simulink model "CHB1"  (R2014b)
settings: Solver=ode23tb  StartTime=0.0  StopTime=0.57  MaxStep=0.0001  RelTol=1e-3
libraries: powerlib x33, RCTblocks x1
settings Model: Creator=selva  LastModifiedBy=SELVA
settings DataIOCC: SignalLoggingSaveFormat=ModelDataLogs
settings OptimizationCC: ExpressionDepthLimit=2147483647
settings DebuggingCC: UnderspecifiedInitializationDetection=Classic  MergeDetectMultiDrivingBlocksExec=none  FcnCallInpInsideContextMsg=UseLocalSettings  StateNameClashWarn=warning
settings GRTTargetCC: CombineOutputUpdateFcns=off  GRTInterface=on

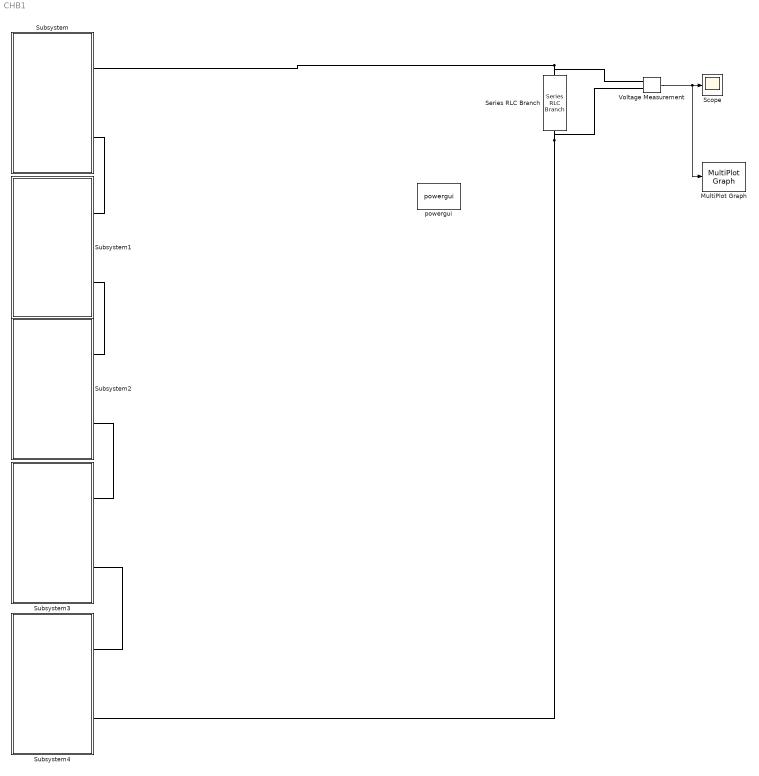
== system CHB1 ==
  MultiPlot Graph : RCTblocks/MultiPlot Graph  Tag=MultiPlot  tmin=0  tmax=20  ymin=-1  ymax=1  Tsamp=-1  vnamesave=multisimout
  Scope : Scope
      settings: YMin=-4e+17  YMax=4e+17
  Series RLC Branch : powerlib/Elements/Series RLC Branch  LConnTagsString=__new0  RConnTagsString=__new0  BranchType=R  Resistance=100  Inductance=1e-3  SetiL0=off  InitialCurrent=0  Capacitance=1e-6  Setx0=off  InitialVoltage=0  Measurements=None
  Subsystem : Subsystem
  Subsystem1 : Subsystem
  Subsystem2 : Subsystem
  Subsystem3 : Subsystem
  Subsystem4 : Subsystem
  Voltage Measurement : powerlib/Measurements/Voltage Measurement  PhasorSimulation=off  OutputType=Complex  PSBequivalent=0
  powergui : powerlib/powergui  Priority=1  SimulationMode=Continuous  SolverType=Tustin/Backward Euler (TBE)  SampleTime=50e-6  frequency=60  SPID=off  DisableSnubberDevices=off  DisableRonSwitches=off  DisableVfSwitches=off  SwTol=0  DisplayEquations=off  Interpol=off  methode=off  Ts=100  frequencyindice=0  Pbase=100e6  ErrMax=1e-4  Iterations=50  UnitsV=kV  UnitsW=MW  FunctionMessages=off  echomessages=off  HookPort=off  EnableUseOfTLC=off  x0status=blocks  RestoreLinks=warning  ResistiveCurrentMeasurement=off  Frange=[0:2:500]  Ylog=off  Xlog=on  ShowGrid=off  save=off  variable=ZData  structure=ScopeData  ZoomFFT=off  StartTime=0.01  cycles=1  DisplayStyle=1  fundamental=50  FreqAxis=off  MaxFrequency=1000  frequencyindicesteady=1  RmsSteady=1  display=off
  wires:
  Voltage Measurement/1 -> MultiPlot Graph/1, Scope/1
  connections:
  Subsystem1/RConn2 -- Subsystem2/RConn1
  Subsystem2/RConn2 -- Subsystem3/RConn1
  Subsystem3/RConn2 -- Subsystem4/RConn1
  Series RLC Branch/LConn1 -- Subsystem/RConn1 -- Voltage Measurement/LConn1
  Series RLC Branch/RConn1 -- Subsystem4/RConn2 -- Voltage Measurement/LConn2
  Subsystem1/RConn1 -- Subsystem/RConn2

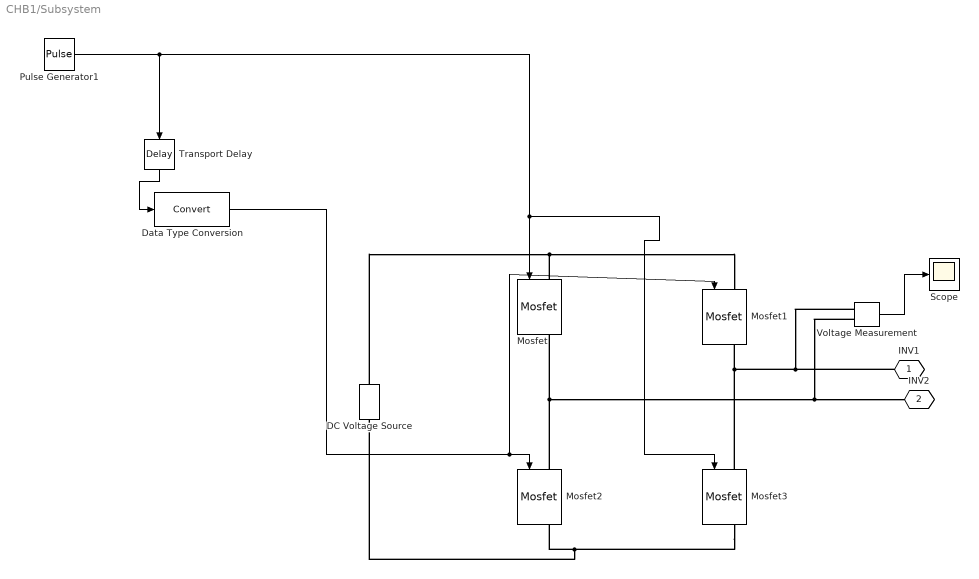
== system CHB1/Subsystem ==
  DC Voltage Source : powerlib/Electrical Sources/DC Voltage Source  Amplitude=65  Measurements=None
  Data Type Conversion : DataTypeConversion
  Mosfet{,1..3} (4 alike) : powerlib/Power Electronics/Mosfet  Ron=0.1  Lon=0  Rd=0.01  Vfd=0  IC=0  Rs=1e5  Cs=inf  Measurements=on
  Pulse Generator1 : DiscretePulseGenerator  PulseType=Time based  Period=.02  PulseWidth=50  PhaseDelay=0.01/11
  Scope : Scope
      settings: YMin=-10  YMax=10
  Transport Delay : TransportDelay  DelayTime=0.01
  Voltage Measurement : powerlib/Measurements/Voltage Measurement  PhasorSimulation=off  OutputType=Complex  PSBequivalent=0
  INV1 : PMIOPort  Tag=PMCPort  Port=1  Side=Right
  INV2 : PMIOPort  Tag=PMCPort  Port=2  Side=Right
  wires:
  Pulse Generator1/1 -> Transport Delay/1, Mosfet3/1, Mosfet/1
  Data Type Conversion/1 -> Mosfet2/1, Mosfet1/1
  Transport Delay/1 -> Data Type Conversion/1
  Voltage Measurement/1 -> Scope/1
  connections:
  Mosfet2/LConn1 -- Mosfet/RConn1 -- Voltage Measurement/LConn2 -- INV2/RConn1
  DC Voltage Source/RConn1 -- Mosfet1/LConn1 -- Mosfet/LConn1
  DC Voltage Source/LConn1 -- Mosfet3/RConn1 -- Mosfet2/RConn1
  Mosfet1/RConn1 -- Voltage Measurement/LConn1 -- INV1/RConn1 -- Mosfet3/LConn1

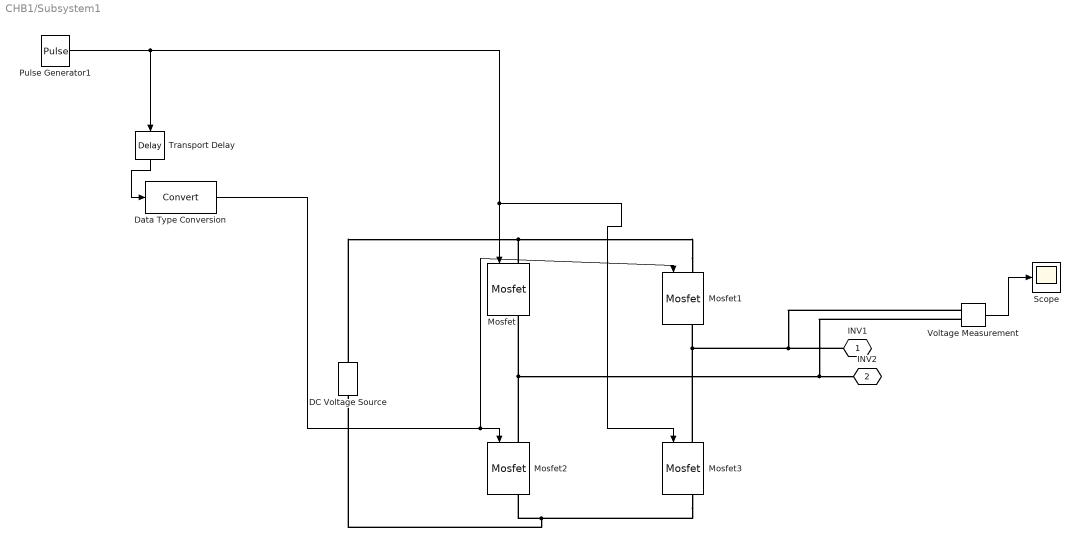
== system CHB1/Subsystem1 ==
  DC Voltage Source : powerlib/Electrical Sources/DC Voltage Source  Amplitude=65  Measurements=None
  Data Type Conversion : DataTypeConversion
  Mosfet{,1..3} (4 alike) : powerlib/Power Electronics/Mosfet  Ron=0.1  Lon=0  Rd=0.01  Vfd=0  IC=0  Rs=1e5  Cs=inf  Measurements=on
  Pulse Generator1 : DiscretePulseGenerator  PulseType=Time based  Period=.02  PulseWidth=50  PhaseDelay=(0.01/11)*2
  Scope : Scope
      settings: YMin=-10  YMax=10  SaveName=ScopeData2
  Transport Delay : TransportDelay  DelayTime=0.01
  Voltage Measurement : powerlib/Measurements/Voltage Measurement  PhasorSimulation=off  OutputType=Complex  PSBequivalent=0
  INV1 : PMIOPort  Tag=PMCPort  Port=1  Side=Right
  INV2 : PMIOPort  Tag=PMCPort  Port=2  Side=Right
  wires:
  Transport Delay/1 -> Data Type Conversion/1
  Data Type Conversion/1 -> Mosfet1/1, Mosfet2/1
  Pulse Generator1/1 -> Mosfet/1, Mosfet3/1, Transport Delay/1
  Voltage Measurement/1 -> Scope/1
  connections:
  INV1/RConn1 -- Voltage Measurement/LConn1 -- Mosfet1/RConn1 -- Mosfet3/LConn1
  Mosfet3/RConn1 -- DC Voltage Source/LConn1 -- Mosfet2/RConn1
  Mosfet1/LConn1 -- DC Voltage Source/RConn1 -- Mosfet/LConn1
  Mosfet/RConn1 -- Voltage Measurement/LConn2 -- INV2/RConn1 -- Mosfet2/LConn1

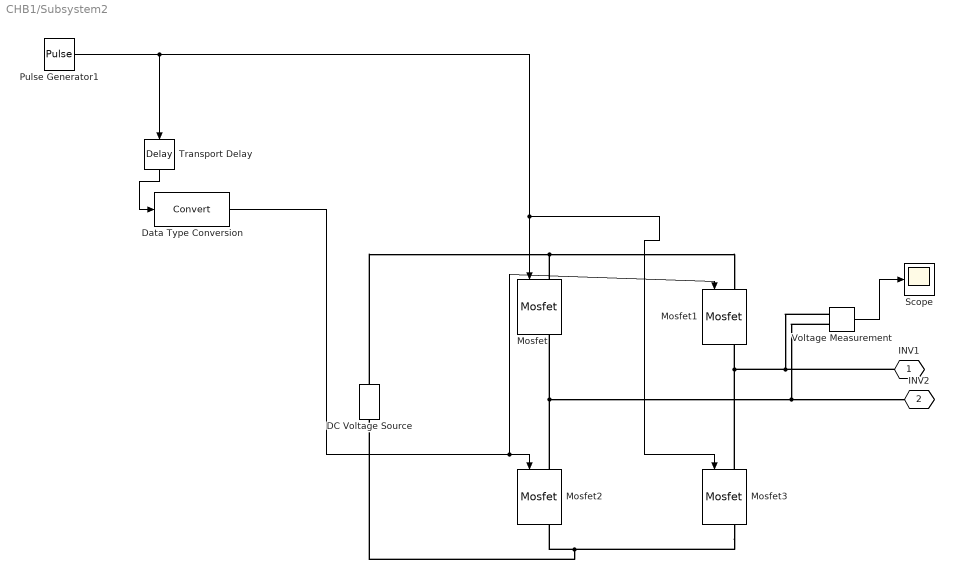
== system CHB1/Subsystem2 ==
  DC Voltage Source : powerlib/Electrical Sources/DC Voltage Source  Amplitude=65  Measurements=None
  Data Type Conversion : DataTypeConversion
  Mosfet{,1..3} (4 alike) : powerlib/Power Electronics/Mosfet  Ron=0.1  Lon=0  Rd=0.01  Vfd=0  IC=0  Rs=1e5  Cs=inf  Measurements=on
  Pulse Generator1 : DiscretePulseGenerator  PulseType=Time based  Period=.02  PulseWidth=50  PhaseDelay=(0.01/11)*3
  Scope : Scope
      settings: YMin=-10  YMax=10  SaveName=ScopeData3
  Transport Delay : TransportDelay  DelayTime=0.01
  Voltage Measurement : powerlib/Measurements/Voltage Measurement  PhasorSimulation=off  OutputType=Complex  PSBequivalent=0
  INV1 : PMIOPort  Tag=PMCPort  Port=1  Side=Right
  INV2 : PMIOPort  Tag=PMCPort  Port=2  Side=Right
  wires:
  Pulse Generator1/1 -> Transport Delay/1, Mosfet3/1, Mosfet/1
  Data Type Conversion/1 -> Mosfet2/1, Mosfet1/1
  Transport Delay/1 -> Data Type Conversion/1
  Voltage Measurement/1 -> Scope/1
  connections:
  Mosfet2/LConn1 -- INV2/RConn1 -- Voltage Measurement/LConn2 -- Mosfet/RConn1
  Mosfet/LConn1 -- DC Voltage Source/RConn1 -- Mosfet1/LConn1
  Mosfet2/RConn1 -- DC Voltage Source/LConn1 -- Mosfet3/RConn1
  Mosfet3/LConn1 -- Voltage Measurement/LConn1 -- INV1/RConn1 -- Mosfet1/RConn1

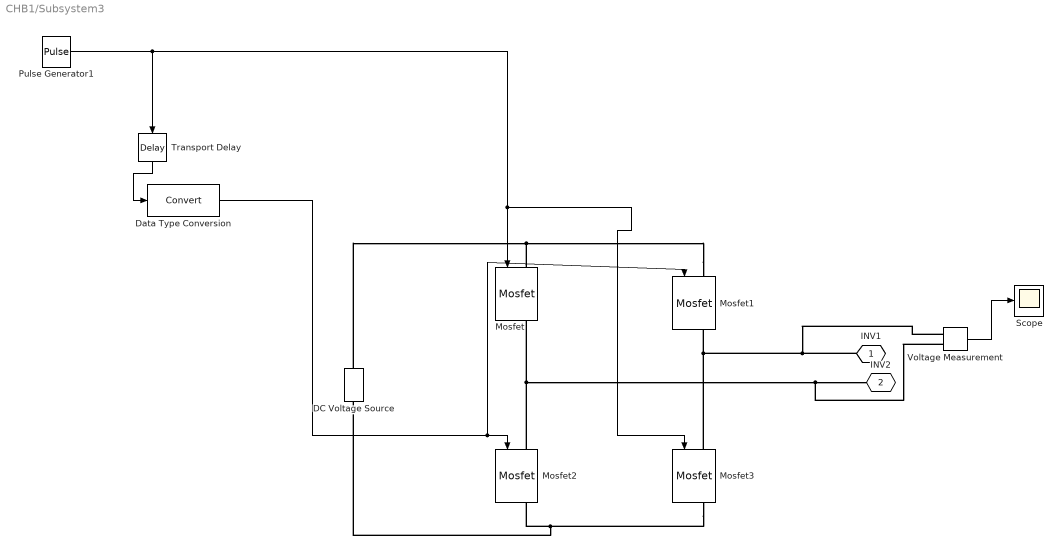
== system CHB1/Subsystem3 ==
  DC Voltage Source : powerlib/Electrical Sources/DC Voltage Source  Amplitude=65  Measurements=None
  Data Type Conversion : DataTypeConversion
  Mosfet{,1..3} (4 alike) : powerlib/Power Electronics/Mosfet  Ron=0.1  Lon=0  Rd=0.01  Vfd=0  IC=0  Rs=1e5  Cs=inf  Measurements=on
  Pulse Generator1 : DiscretePulseGenerator  PulseType=Time based  Period=0.02  PulseWidth=50  PhaseDelay=(0.01/11)*4
  Scope : Scope
      settings: YMin=-10  YMax=10  SaveName=ScopeData4
  Transport Delay : TransportDelay  DelayTime=0.01
  Voltage Measurement : powerlib/Measurements/Voltage Measurement  PhasorSimulation=off  OutputType=Complex  PSBequivalent=0
  INV1 : PMIOPort  Tag=PMCPort  Port=1  Side=Right
  INV2 : PMIOPort  Tag=PMCPort  Port=2  Side=Right
  wires:
  Transport Delay/1 -> Data Type Conversion/1
  Data Type Conversion/1 -> Mosfet1/1, Mosfet2/1
  Pulse Generator1/1 -> Mosfet/1, Mosfet3/1, Transport Delay/1
  Voltage Measurement/1 -> Scope/1
  connections:
  INV1/RConn1 -- Voltage Measurement/LConn1 -- Mosfet1/RConn1 -- Mosfet3/LConn1
  Mosfet3/RConn1 -- DC Voltage Source/LConn1 -- Mosfet2/RConn1
  Mosfet1/LConn1 -- DC Voltage Source/RConn1 -- Mosfet/LConn1
  Mosfet/RConn1 -- Voltage Measurement/LConn2 -- INV2/RConn1 -- Mosfet2/LConn1

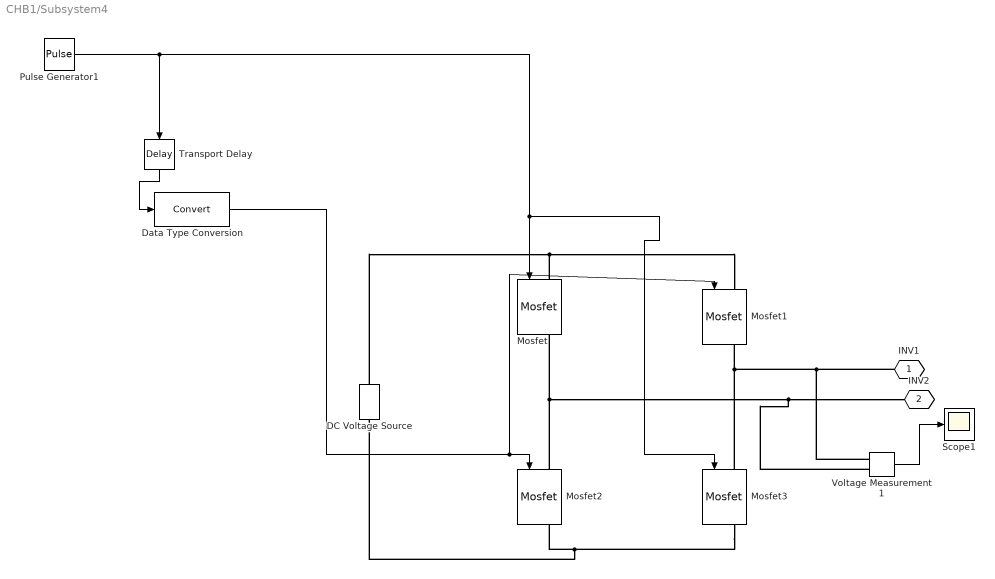
== system CHB1/Subsystem4 ==
  DC Voltage Source : powerlib/Electrical Sources/DC Voltage Source  Amplitude=65  Measurements=None
  Data Type Conversion : DataTypeConversion
  Mosfet{,1..3} (4 alike) : powerlib/Power Electronics/Mosfet  Ron=0.1  Lon=0  Rd=0.01  Vfd=0  IC=0  Rs=1e5  Cs=inf  Measurements=on
  Pulse Generator1 : DiscretePulseGenerator  PulseType=Time based  Period=.02  PulseWidth=50  PhaseDelay=(0.01/11)*5
  Scope1 : Scope
      settings: YMin=-10  YMax=10  SaveName=ScopeData6
  Transport Delay : TransportDelay  DelayTime=0.01
  Voltage Measurement1 : powerlib/Measurements/Voltage Measurement  PhasorSimulation=off  OutputType=Complex  PSBequivalent=0
  INV1 : PMIOPort  Tag=PMCPort  Port=1  Side=Right
  INV2 : PMIOPort  Tag=PMCPort  Port=2  Side=Right
  wires:
  Pulse Generator1/1 -> Transport Delay/1, Mosfet3/1, Mosfet/1
  Data Type Conversion/1 -> Mosfet2/1, Mosfet1/1
  Transport Delay/1 -> Data Type Conversion/1
  Voltage Measurement1/1 -> Scope1/1
  connections:
  Mosfet2/LConn1 -- Voltage Measurement1/LConn2 -- INV2/RConn1 -- Mosfet/RConn1
  Mosfet/LConn1 -- DC Voltage Source/RConn1 -- Mosfet1/LConn1
  Mosfet2/RConn1 -- DC Voltage Source/LConn1 -- Mosfet3/RConn1
  Mosfet3/LConn1 -- Voltage Measurement1/LConn1 -- INV1/RConn1 -- Mosfet1/RConn1
